simulink model "maglev"  (R2015a)
settings: Solver=ode45  StartTime=0.0  StopTime=5  RelTol=1e-3
values from neighbouring files (symbols this model uses):
  Astar = zeros(3,3,9)    [magnetic_lev.m]
  dstar = zeros(3,9)    [magnetic_lev.m]
  g = 9.81    [magnetic_lev.m]
  hdot_start = 0    [magnetic_lev.m]
  hmax = 0.07    [magnetic_lev.m]
  hmin = 0.03    [magnetic_lev.m]
  hstart = 0.03    [magnetic_lev.m]
  imax = 3    [magnetic_lev.m]
  imin = 0.1    [magnetic_lev.m]
  istart = 0    [magnetic_lev.m]
  K = zeros(9,4)    [magnetic_lev.m]
  Km = km/m    (= 0.01029)    [magnetic_lev.m]
  L = 10^-5    (= 1e-05)    [magnetic_lev.m]
  R = 0.92    [magnetic_lev.m]
libraries: fuzblock x1
settings Model: NumberOfSteps=100  Creator=Charilaos  LastModifiedBy=Charilaos

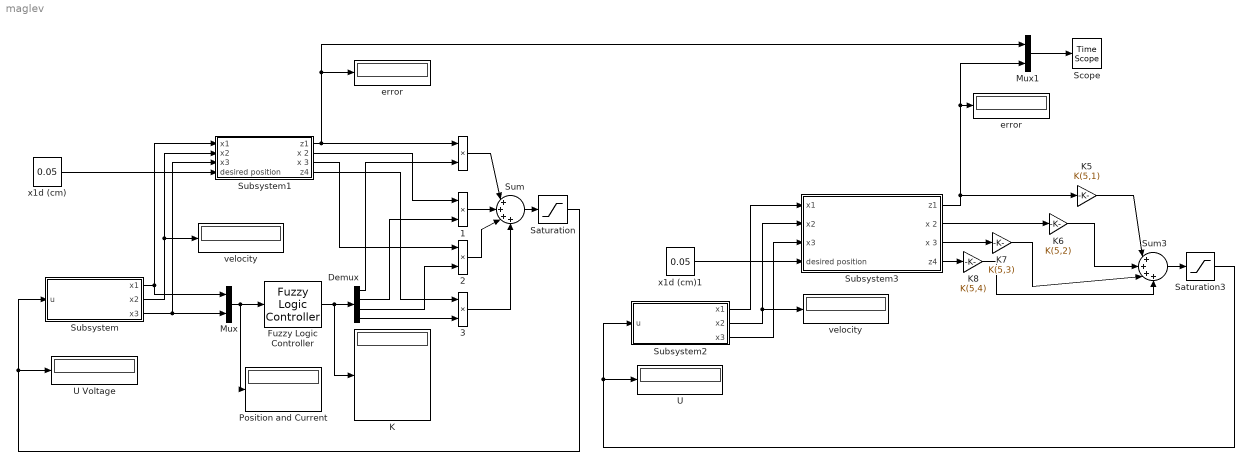
== system maglev ==
   {,1..3} (4 alike) : Product
  Demux : Demux
  Fuzzy Logic Controller : fuzblock/Fuzzy Logic  Controller  fis='sugeno.fis'
  K : Display
  K5 : Gain  Gain=K(5,1)
  K6 : Gain  Gain=K(5,2)
  K7 : Gain  Gain=K(5,3)
  K8 : Gain  Gain=K(5,4)
  Mux : Mux  Inputs=2
  Mux1 : Mux  Inputs=2
  Position and Current : Display
  Saturation : Saturate  UpperLimit=5  LowerLimit=-5  ZeroCross=off
  Saturation3 : Saturate  UpperLimit=5  LowerLimit=0
  "Scope " : TimeScope
  Subsystem : Subsystem
  Subsystem1 : Subsystem
  Subsystem2 : Subsystem
  Subsystem3 : Subsystem
  Sum : Sum  Inputs=|++++
  Sum3 : Sum  Inputs=|++++
  "U " : Display
  U Voltage : Display
  error : Display
  "error " : Display
  velocity : Display
  "velocity " : Display
  x1d (cm) : Constant  Value=0.05
  x1d (cm)1 : Constant  Value=0.05
  wires:
  Mux/1 -> Position and Current/1, Fuzzy Logic Controller/1
  Subsystem/1(x1) -> Subsystem1/1(x1), Mux/1
  Subsystem/3(x3) -> Subsystem1/3(x3), Mux/2
  Subsystem/2(x2) -> velocity/1, Subsystem1/2(x2)
  Demux/3 -> " 2"/2
  Fuzzy Logic Controller/1 -> K/1, Demux/1
  Demux/1 -> " "/2
  Demux/2 -> " 1"/2
  Demux/4 -> " 3"/2
  " "/1 -> Sum/1
  " 1"/1 -> Sum/2
  " 2"/1 -> Sum/3
  " 3"/1 -> Sum/4
  x1d (cm)/1 -> Subsystem1/4(desired position)
  Sum/1 -> Saturation/1
  Subsystem1/1(z1) -> " "/1, Mux1/1, error/1
  Subsystem1/2(x 2) -> " 1"/1
  Subsystem1/3(x 3) -> " 2"/1
  Subsystem1/4(z4) -> " 3"/1
  Saturation/1 -> U Voltage/1, Subsystem/1(u)
  Sum3/1 -> Saturation3/1
  K5/1 -> Sum3/1
  K6/1 -> Sum3/2
  K7/1 -> Sum3/3
  K8/1 -> Sum3/4
  Mux1/1 -> "Scope "/1
  Subsystem2/1(x1) -> Subsystem3/1(x1)
  Subsystem2/3(x3) -> Subsystem3/3(x3)
  Subsystem2/2(x2) -> "velocity "/1, Subsystem3/2(x2)
  x1d (cm)1/1 -> Subsystem3/4(desired position)
  Subsystem3/1(z1) -> K5/1, Mux1/2, "error "/1
  Subsystem3/2(x 2) -> K6/1
  Subsystem3/3(x 3) -> K7/1
  Subsystem3/4(z4) -> K8/1
  Saturation3/1 -> Subsystem2/1(u), "U "/1

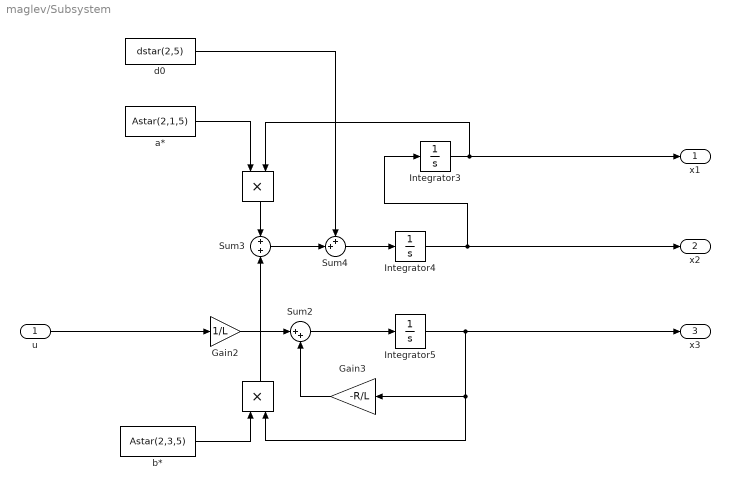
== system maglev/Subsystem ==
  u : Inport
  " " : Product
  "  " : Product
  Gain2 : Gain  Gain=1/L
  Gain3 : Gain  Gain=-R/L
  Integrator3 : Integrator  InitialCondition=hstart  LimitOutput=on  UpperSaturationLimit=hmax  LowerSaturationLimit=hmin
  Integrator4 : Integrator  InitialCondition=hdot_start  UpperSaturationLimit=9.81
  Integrator5 : Integrator  InitialCondition=istart  UpperSaturationLimit=imax  LowerSaturationLimit=imin
  Sum2 : Sum  Inputs=|++
  Sum3 : Sum  Inputs=+|+
  Sum4 : Sum  Inputs=++|
  a* : Constant  Value=Astar(2,1,5)
  b* : Constant  Value=Astar(2,3,5)
  "d0 " : Constant  Value=dstar(2,5)
  x1 : Outport
  x2 : Outport  Port=2
  x3 : Outport  Port=3
  wires:
  Integrator3/1 -> x1/1, "  "/2
  Integrator4/1 -> Integrator3/1, x2/1
  Integrator5/1 -> x3/1, " "/2, Gain3/1
  Gain2/1 -> Sum2/1
  Gain3/1 -> Sum2/2
  Sum2/1 -> Integrator5/1
  "  "/1 -> Sum3/1
  " "/1 -> Sum3/2
  u/1 -> Gain2/1
  Sum3/1 -> Sum4/2
  Sum4/1 -> Integrator4/1
  a*/1 -> "  "/1
  "d0 "/1 -> Sum4/1
  b*/1 -> " "/1

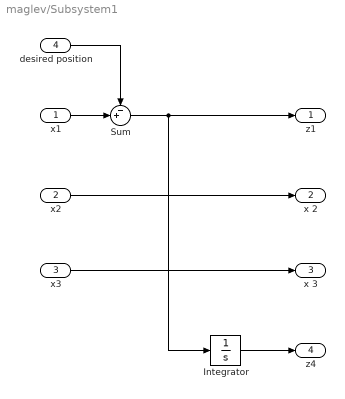
== system maglev/Subsystem1 ==
  x1 : Inport
  x2 : Inport  Port=2
  x3 : Inport  Port=3
  desired position : Inport  Port=4
  Integrator : Integrator
  Sum : Sum  Inputs=-+|
  z1 : Outport
  x 2 : Outport  Port=2
  x 3 : Outport  Port=3
  z4 : Outport  Port=4
  wires:
  x2/1 -> x 2/1
  x3/1 -> x 3/1
  x1/1 -> Sum/2
  desired position/1 -> Sum/1
  Sum/1 -> Integrator/1, z1/1
  Integrator/1 -> z4/1

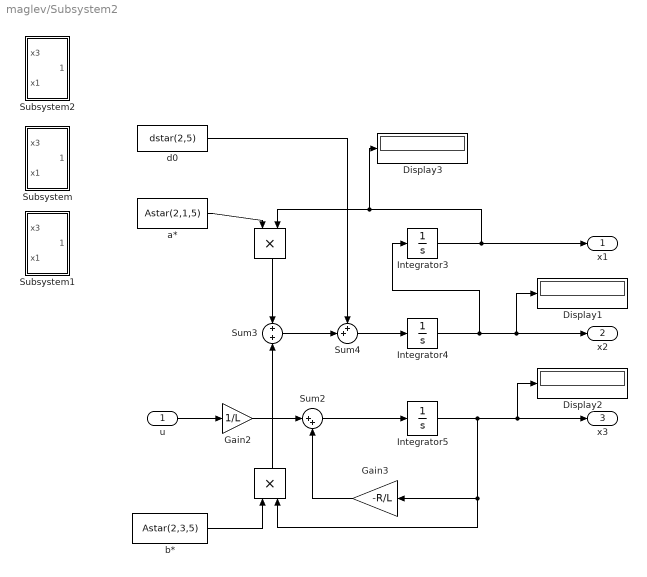
== system maglev/Subsystem2 ==
  u : Inport
  " " : Product
  "  " : Product
  Display1 : Display
  Display2 : Display
  Display3 : Display
  Gain2 : Gain  Gain=1/L
  Gain3 : Gain  Gain=-R/L
  Integrator3 : Integrator  InitialCondition=hstart  LimitOutput=on  UpperSaturationLimit=hmax  LowerSaturationLimit=hmin
  Integrator4 : Integrator  InitialCondition=hdot_start  UpperSaturationLimit=9.81
  Integrator5 : Integrator  InitialCondition=istart  UpperSaturationLimit=imax  LowerSaturationLimit=imin
  Subsystem : Subsystem
  Subsystem1 : Subsystem
  Subsystem2 : Subsystem
  Sum2 : Sum  Inputs=|++
  Sum3 : Sum  Inputs=+|+
  Sum4 : Sum  Inputs=++|
  a* : Constant  Value=Astar(2,1,5)
  b* : Constant  Value=Astar(2,3,5)
  "d0 " : Constant  Value=dstar(2,5)
  x1 : Outport
  x2 : Outport  Port=2
  x3 : Outport  Port=3
  wires:
  Integrator3/1 -> x1/1, Display3/1, "  "/2
  Integrator4/1 -> Integrator3/1, x2/1, Display1/1
  Integrator5/1 -> x3/1, Display2/1, " "/2, Gain3/1
  Gain2/1 -> Sum2/1
  Gain3/1 -> Sum2/2
  Sum2/1 -> Integrator5/1
  "  "/1 -> Sum3/1
  " "/1 -> Sum3/2
  u/1 -> Gain2/1
  Sum3/1 -> Sum4/2
  Sum4/1 -> Integrator4/1
  a*/1 -> "  "/1
  "d0 "/1 -> Sum4/1
  b*/1 -> " "/1

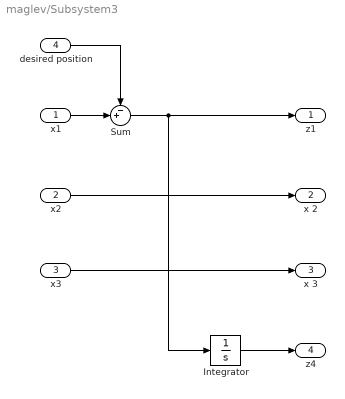
== system maglev/Subsystem3 ==
  x1 : Inport
  x2 : Inport  Port=2
  x3 : Inport  Port=3
  desired position : Inport  Port=4
  Integrator : Integrator
  Sum : Sum  Inputs=-+|
  z1 : Outport
  x 2 : Outport  Port=2
  x 3 : Outport  Port=3
  z4 : Outport  Port=4
  wires:
  x2/1 -> x 2/1
  x3/1 -> x 3/1
  x1/1 -> Sum/2
  desired position/1 -> Sum/1
  Sum/1 -> Integrator/1, z1/1
  Integrator/1 -> z4/1

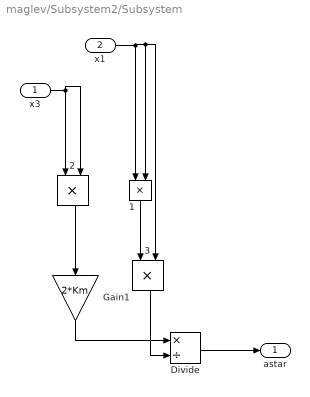
== system maglev/Subsystem2/Subsystem ==
  x3 : Inport
  "x1 " : Inport  Port=2
  "  1" : Product
  "  2" : Product
  "  3" : Product
  Divide : Product  Inputs=*/
  Gain1 : Gain  Gain=2*Km
  astar : Outport
  wires:
  x3/1 -> "  2"/1, "  2"/2
  "  3"/1 -> Divide/2
  Divide/1 -> astar/1
  Gain1/1 -> Divide/1
  "  2"/1 -> Gain1/1
  "x1 "/1 -> "  1"/1, "  3"/2, "  1"/2
  "  1"/1 -> "  3"/1

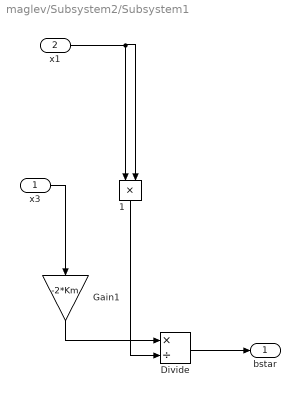
== system maglev/Subsystem2/Subsystem1 ==
  x3 : Inport
  "x1 " : Inport  Port=2
  "  1" : Product
  Divide : Product  Inputs=*/
  Gain1 : Gain  Gain=-2*Km
  "bstar " : Outport
  wires:
  "  1"/1 -> Divide/2
  Divide/1 -> "bstar "/1
  Gain1/1 -> Divide/1
  x3/1 -> Gain1/1
  "x1 "/1 -> "  1"/1, "  1"/2

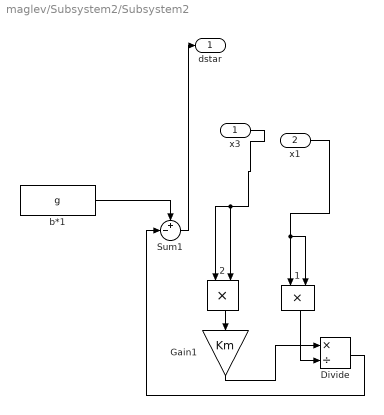
== system maglev/Subsystem2/Subsystem2 ==
  x3 : Inport
  x1 : Inport  Port=2
  "  1" : Product
  "  2" : Product
  Divide : Product  Inputs=*/
  Gain1 : Gain  Gain=Km
  Sum1 : Sum  Inputs=+-|
  b*1 : Constant  Value=g
  "dstar " : Outport
  wires:
  x3/1 -> "  2"/1, "  2"/2
  x1/1 -> "  1"/2, "  1"/1
  Gain1/1 -> Divide/1
  "  1"/1 -> Divide/2
  Divide/1 -> Sum1/2
  "  2"/1 -> Gain1/1
  b*1/1 -> Sum1/1
  Sum1/1 -> "dstar "/1
